simulink library "SimFly_Sensors"  (R2015b)
settings: Solver=VariableStepAuto  StartTime=0.0  StopTime=10.0  RelTol=1e-3
(part 1 of 2)
settings Model: Creator=mocherma  LastModifiedBy=mocherma

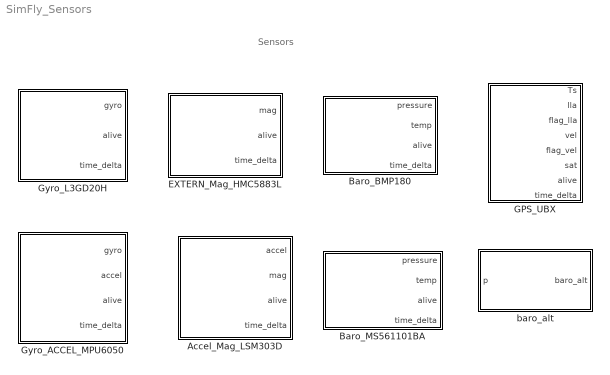
== system SimFly_Sensors ==
  note: Sensors
  Accel_Mag_LSM303D : MATLAB Function  TreatAsAtomicUnit=on  mask(SimFly Accel Magnetometer){sA0=HIGH, ascale=2G, lowPassFreq=773Hz, mscale=-/+ 2 gauss, rate=50Hz, lsm303d_sample_time=-1}
      mask prompts: ascale "Accel Scale"; lowPassFreq "Low Pass Cut-Off Frequency"; mscale "Mag Scale"; rate "Output Rate"; lsm303d_sample_time "SampleTime"
      mask help:
      | LSM303 MEMS motion sensor: 3-axis accelerometer and 3-axis magnetometer
      | Accelerometer full-scale range of ±2 g/±4 g/±8 g
      | Magnetometer ±1.3 to ±8,1 gauss magnetic field full-scale
      |
      | ...........Caution!................
      |
      | If External Magnetometer HMC5883L is in use SA0 must be
      |
      | HIGH due to the same I2C Address.
      |
      | ....................
      |
      | All quantities are in body axes. Signs are as follows:
      | +ax [rad/s]
      | +ay [rad/s]
      | +az [rad/s]
      | +mx [gauss]
      | +my [gauss]
      | +mz [gauss]
      |
      | Inputs are to pass through data when in simulation mode.
      | They are not used when model is deployed to hardware.
      |
      | Execution Time: 465 µS
      mask init:
      | sA0;
      | blk = gcb;
      | sA0String = get_param(blk,'sA0');
      | if strcmp(sA0String,'HIGH');
      |     sA0Pin = true;
      | else sA0Pin = false;
      | end
      | 
      | scaleaccString =get_param(blk,'ascale');
      | switch scaleaccString
      |     case '2G'
      |         scaleAc= uint8(0);
      |     case '4G'
      |         scaleAc= uint8(1);
      |     case '6G'
      |         scaleAc= uint8(2);
      |     case '8G'
      |         scaleAc= uint8(3);
      |     case '16G'
      |         scaleAc= uint8(4);
      |     otherwise
      |         scaleAc= uint8(0);
      | end
      | scalemagString =get_param(blk,'mscale');
      | switch scalemagString
      |     case '-/+ 2 gauss'
      |         scaleMag= uint8(0);
      |     case '-/+ 4 gauss'
      |         scaleMag= uint8(1);
      |     case '-/+ 8 gauss'
      |         scaleMag= uint8(2);
      |     case '-/+ 12 gauss'
      |         scaleMag= uint8(3);    
      |     otherwise
      |         scaleMag= uint8(1);
      | end        
      | lowPassString =get_param(blk,'lowPassFreq');
      | switch lowPassString
      |     case '773Hz'
      |         lowPassFreq= uint8(0);
      |     case '362Hz'
      |         lowPassFreq= uint8(1);
      |     case '194Hz'
      |         lowPassFreq= uint8(2);
      |     case '50Hz'
      |         lowPassFreq= uint8(3);    
      |     otherwise
      |         lowPassFreq= uint8(0);
      | end        
      | rateString =get_param(blk,'rate');
      | switch rateString
      |     case '50Hz'
      |         rateVal= uint8(0);
      |     case '100Hz'
      |         rateVal= uint8(1);
      |     case '200Hz'
      |         rateVal= uint8(2);
      |     case '400Hz'
      |         rateVal= uint8(3);
      |     otherwise
      |         rateVal= uint8(3);
      | end
  Baro_BMP180 : MATLAB Function  TreatAsAtomicUnit=on  mask(SimFly Barometer){osr=4.5ms, bmp180_sample_time=-1}
      mask prompts: osr "Oversampling Time"; bmp180_sample_time "Sample Time"
      mask help:
      | BMP180 DIGITAL PRESSURE SENSOR
      | Measures Pressure (mb)
      | Signs are as follows:
      | +p [mb]
      |
      | Oversampling Ratio: delay time for sampling measurements
      | 4.5ms / 7.5ms / 13.5ms / 25.5ms
      |
      | ........Caution......
      |
      | If used with Baro_MS5611 Baros's SD0 must be High
      |
      | .....................
      |
      |
      | Inputs are to pass through data when in simulation mode.
      | They are not used when model is deployed to hardware.
      |
      | Execution Time: 350µS
      mask init:
      | blk = gcb;
      | scaleString =get_param(blk,'osr');
      | switch scaleString
      |     case '4.5ms'
      |         osrValue= uint8(0);
      |     case '7.5ms'
      |         osrValue= uint8(1);
      |     case '13.5ms'
      |         osrValue= uint8(2);
      |     case '25.5ms'
      |         osrValue= uint8(3);        
      |     otherwise
      |         osrValue= uint8(0);
      | end
  Baro_MS561101BA : MATLAB Function  TreatAsAtomicUnit=on  mask(SimFly Barometer){sD0=LOW, osr=256, ms5611_sample_time=-1}
      mask prompts: osr "Oversampling Ratio"; ms5611_sample_time "Sample Time"
      mask help:
      | MS5611 DIGITAL PRESSURE SENSOR
      | Measures Pressure (mb)
      |
      | ...........Caution!................
      |
      | If  BMP180 is in use SD0 must be
      |
      | HIGH due to the same I2C Address.
      |
      | ...................................
      |
      |
      | Oversampling Ratio: delay time for sampling measurements
      | 256     =   1ms
      | 512     =   2ms
      | 1024    =   3ms
      | 2048    =   5ms
      | 4096    =   10ms
      |
      | Signs are as follows:
      | +p [mb]
      |
      | Inputs are to pass through data when in simulation mode.
      | They are not used when model is deployed to hardware.
      |
      | Execution Time: 600µS
      mask init:
      | sD0;
      | blk = gcb;
      | sD0String = get_param(blk,'sD0');
      | if strcmp(sD0String,'HIGH');
      |     sD0Pin = true;
      | else sD0Pin = false;
      | end
      | 
      | scaleString =get_param(blk,'osr');
      | switch scaleString
      |     case '256'
      |         osrValue= uint8(0);
      |     case '512'
      |         osrValue= uint8(1);
      |     case '1024'
      |         osrValue= uint8(2);
      |     case '2048'
      |         osrValue= uint8(3);
      |     case '4096'
      |         osrValue= uint8(4);          
      |     otherwise
      |         osrValue= uint8(1);
      | end
  EXTERN_Mag_HMC5883L : MATLAB Function  TreatAsAtomicUnit=on  mask(SimFly Magnetometer){range=+/- 0.88 Ga, rate=0.75Hz, samples=1, hmc_sample_time=-1}
      mask prompts: range "Sensor Field Range"; rate "Data Output Rate (Hz)"; samples "Number of samples averaged"; hmc_sample_time "Sample Time"
      mask help:
      | Honeywell HMC5883L MEMS 3-Axis Digital Compass
      | Magnetometer ±0.88 to ±8,1 gauss magnetic field full-scale
      | Output rate from 0.75Hz to 75Hz
      | Select number of samples averaged (1 to 8) per measurement output.
      |
      | ........Caution......
      |
      | If used with Accel LSM303 Accels's AD0 must be High
      |
      | .....................
      |
      | Inputs are to pass through data when in simulation mode.
      | They are not used when model is deployed to hardware.
      |
      | Execution Time: 555 µS
      mask init:
      | blk = gcb;
      | 
      | rangeString = get_param(blk,'range');
      | switch rangeString
      |     case '+/- 0.88 Ga'
      |         rangeString= uint8(1);
      |     case '+/-   1.3 Ga'
      |         rangeString= uint8(2);
      |     case '+/-   1.9 Ga'
      |         rangeString= uint8(3);
      |     case '+/-   2.5 Ga'
      |         rangeString= uint8(4);
      |     case '+/-   4.0 Ga'
      |         rangeString= uint8(5);
      |     case '+/-   4.7 Ga'
      |         rangeString= uint8(6);
      |     case '+/-   5.6 Ga'
      |         rangeString= uint8(7);
      |     case '+/-   8.1 Ga'
      |         rangeString= uint8(8);
      |     otherwise
      |         rangeString= uint8(1);
      | end
      | 
      | rateString =get_param(blk,'rate');
      | switch rateString
      |     case '0.75Hz'
      |         rateString= uint8(0);
      |     case '1.5Hz'
      |         rateString= uint8(1);
      |     case '3Hz'
      |         rateString= uint8(2);
      |     case '7.5Hz'
      |         rateString= uint8(3);
      |     case '15Hz'
      |         rateString= uint8(4);
      |     case '30Hz'
      |         rateString= uint8(5);
      |     case '75Hz'
      |         rateString= uint8(6);
      |     otherwise
      |         rateString= uint8(4);
      | end
      | 
      | 
      | samplesString =get_param(blk,'samples');
      | switch samplesString
      |     case '1'
      |         samplesString= uint8(0);
      |     case '2'
      |         samplesString= uint8(1);
      |     case '4'
      |         samplesString= uint8(2);
      |     case '8'
      |         samplesString= uint8(3);
      |     otherwise
      |         samplesString= uint8(0);
      | end
  GPS_UBX : MATLAB Function  TreatAsAtomicUnit=on  mask(SimFly GNSS){ubx_sample_time=-1}
      mask prompts: ubx_sample_time "Sample Time"
      mask help:
      | Block for parsing UMX data streams provided by GPS modules from Ublox.
      |
      | If using LEA-6H:
      | Max. Navigation update rate 5Hz
      |
      |
      | Ouput:
      | - Timestamp
      | - Latitude / Longitude [deg] / Altitude [m]
      | - LLA update flag
      | - ECEF velocity [m/s]
      | - vel update flag
      | - Number of visible satelites
      | - Alive flag
      | - Execution time
  Gyro_ACCEL_MPU6050 : MATLAB Function  TreatAsAtomicUnit=on  mask(SimFly IMU){AD0=HIGH, rate=50Hz, freqMp=5Hz, scaleAcc=2G, scaleGy=250DPS, mpuSampleTime=-1}
      mask prompts: rate "Output Rate"; freqMp "Lowpass Filter Cut Off Freq"; scaleAcc "Accel Scale"; scaleGy "Gyro Scale"; mpuSampleTime "Sample Time"
      mask help:
      | MPU-6050 device combines a 3-axis gyroscope and a 3-axis accelerometer
      | Gyro full-scale range of ±250, ±500, ±1000, and ±2000°/sec
      | Accelerometer full-scale range of ±2g, ±4g, ±8g, and ±16g.
      | All quantities are in body axes. Signs are as follows:
      | +p [rad/s]
      | +q [rad/s]
      | +r [rad/s]
      | +ax [m/s^2]
      | +ay [m/s^2]
      | +az [m/s^2]
      |
      | Inputs are to pass through data when in simulation mode.
      | They are not used when model is deployed to hardware.
      |
      | Execution Time: 464 µS
      mask init:
      | blk = gcb;
      | AD0;
      | AD0String = get_param(blk,'AD0');
      | if strcmp(AD0String,'HIGH');
      |     AD0Pin = true;
      | else AD0Pin = false;
      | end
      | scaleAccel =get_param(blk,'scaleAcc');
      | switch scaleAccel
      |     case '2G'
      |         scaleAccel= uint8(2);
      |     case '4G'
      |         scaleAccel= uint8(4);
      |     case '8G'
      |         scaleAccel= uint8(8);
      |     case '16G'
      |         scaleAccel= uint8(16);
      |     otherwise
      |         scaleAccel= uint8(2);
      | end
      | freqMpu =get_param(blk,'freqMp');
      | switch freqMpu
      |     case '5Hz'
      |         freqMpu= uint8(6);
      |     case '10Hz'
      |         freqMpu= uint8(5);
      |     case '21Hz'
      |         freqMpu= uint8(4);
      |     case '44Hz'
      |         freqMpu= uint8(3);
      |     case '94Hz'
      |         freqMpu= uint8(2);
      |     case '184Hz'
      |         freqMpu= uint8(1);
      |     otherwise
      |         freqMpu= uint8(1);
      | end    
      | 
      | scaleGyro =get_param(blk,'scaleGy');
      | switch scaleGyro
      |     case '250DPS'
      |         scaleGyro= int16(250);
      |     case '500DPS'
      |         scaleGyro= int16(500);
      |     case '1000DPS'
      |         scaleGyro= int16(1000);
      |     case '2000DPS'
      |         scaleGyro= int16(2000);
      |     otherwise
      |         scaleGyro= int16(250);
      | end  
      | 
      | rateString =get_param(blk,'rate');
      | switch rateString
      |     case '50Hz'
      |         rateVal= uint8(19);
      |     case '100Hz'
      |         rateVal= uint8(5);
      |     case '200Hz'
      |         rateVal= uint8(4);
      |     case '250Hz'
      |         rateVal= uint8(3);
      |     case '500Hz'
      |         rateVal= uint8(1);
      |     otherwise
      |         rateVal= uint8(3);
      | end
  Gyro_L3GD20H : MATLAB Function  TreatAsAtomicUnit=on  mask(SimFly Gyro){sD0=HIGH, scale=250DPS, freq=100Hz 12.5 Cut-Off[Hz], l3gd20_sampletime=-1}
      mask prompts: freq "Output Rate + Cutoff Freq"; l3gd20_sampletime "Sample Time"
      mask help:
      | L3GD20 MEMS motion sensor: 3-axis digital gyroscope
      | Gyro full-scale range of ±250, ±500 and ±2000°/sec
      | All quantities are in body axes. Signs are as follows:
      | +p [rad/s]
      | +q [rad/s]
      | +r [rad/s]
      |
      | Inputs are to pass through data when in simulation mode.
      | They are not used when model is deployed to hardware.
      |
      | Execution Time: 234 µS
      mask init:
      | sD0;
      | blk = gcb;
      | sD0String = get_param(blk,'sD0');
      | if strcmp(sD0String,'HIGH');
      |     sD0Pin = true;
      | else sD0Pin = false;
      | end
      | 
      | scaleString =get_param(blk,'scale');
      | switch scaleString
      |     case '250DPS'
      |         scaleValue= uint8(0);
      |     case '500DPS'
      |         scaleValue= uint8(1);
      |     case '2000DPS'
      |         scaleValue= uint8(2);
      |     otherwise
      |         scaleValue= uint8(1);
      | end
      | 
      | freqString =get_param(blk,'freq');
      | switch scaleString
      |     case '100Hz 12.5 Cut-Off[Hz]'
      |         freqValue= uint8(0);
      |     case '100Hz 25 Cut-Off[Hz]'
      |         freqValue= uint8(1);
      |     case '200Hz 0 Cut-Off[Hz]'
      |         freqValue= uint8(2);
      |     case '200Hz 12.5 Cut-Off[Hz]'
      |         freqValue= uint8(3);
      |     case '200Hz 70 Cut-Off[Hz]'
      |         freqValue= uint8(4);
      |     case '400Hz 20 Cut-Off[Hz]'
      |         freqValue= uint8(5);
      |     case '400Hz 50 Cut-Off[Hz]'
      |         freqValue= uint8(6);
      |     case '400Hz 110 Cut-Off[Hz]'
      |         freqValue= uint8(7);
      |     case '800Hz 30 Cut-Off[Hz]'
      |         freqValue= uint8(8);
      |     case '800Hz 100 Cut-Off[Hz]'
      |         freqValue= uint8(9);
      |     otherwise
      |         freqValue= uint8(2);    
      | end
  baro_alt : MATLAB Function  TreatAsAtomicUnit=on  mask(SimFly Barometer Altitude){p0=1013.25, alt_sample_time=-1}
      mask prompts: p0 "Pressure sea level"; alt_sample_time "Sample Time"
      mask help: Calculates the altitude above sea level with a given pressure at sea level in hPa

== matlab function SimFly_Sensors/Gyro_ACCEL_MPU6050 ==
  settings: updateMethod=DISCRETE  sampleTime=mpuSampleTime
  data: gyro output; accel output; alive output; time_delta output; AD0Pin parameter; freqMpu parameter; rateVal parameter; scaleGyro parameter; scaleAccel parameter
function [gyro,accel,alive,time_delta] = MPU6050(  AD0Pin, freqMpu, rateVal, scaleGyro, scaleAccel)
% Simulink Arduino Block Driver Library for Autocode Generation
 % 
 % This file is part of the Simulink Arduino Block Driver Library 
 % for Autocode Generation with Simulink
 %
 % This Library is free software: you can redistribute it and/or modify
 % it under the terms of the GNU General Public License as published by
 % the Free Software Foundation, either version 3 of the License, or
 % (at your option) any later version.
 %
 % This Library is distributed in the hope that it will be useful,
 % but WITHOUT ANY WARRANTY; without even the implied warranty of
 % MERCHANTABILITY or FITNESS FOR A PARTICULAR PURPOSE.  See the
 % GNU General Public License for more details.
 %
 % You should have received a copy of the GNU General Public License
 % along with this Library.  If not, see
 % <http://www.gnu.org/licenses/>.
 %
%
%PURMPOSE: Driver for MPU6050 with hardware abstraction layer
%AUTHOR: Marcell Mocher
%DATE: 10.6.2016
%VERSION: 0.1 V Fist build
%Input: -
%Output:    gyro[3*1](single) =  angular rates in X,Y,Z Axis [rad/s]
%           accel[3*1](single) = acceleration in X,Y,Z Axis [ms^-2]
%           alive(boolean) = boolean if sensor is alive
%           time_delta(single) = time needed to execute funtion [us]
%Info: This drive requires function call triggered simuluink functions in
% order to work
%Requires:  _get_time
%           _serial_init
%           _serial_print
%           _serial_write
%           _i2c_write_register
%           _i2c_read_register

persistent init_flag alive_flag MPU6050_ADDR gyroRes accelRes MPU6050_WHO_AM_I MPU6050_PWR_MGMT_1 MPU6050_CONFIG MPU6050_SMPLRT_DIV ...
    MPU6050_INT_ENABLE MPU6050_GYRO_CONFIG MPU6050_ACCEL_CONFIG MPU6050_GYRO_XOUT_H MPU6050_ACCEL_XOUT_H MPU6050_INT_PIN_CFG;


if strcmp(coder.target, 'rtw'),
    
    time_start = uint32(0);
    time_start = coder.ceval('_get_time');
    
    gyro = single(zeros(3,1));
    accel = single(zeros(3,1));
    
    %Parameter from Mask!
    debug = false;
    
    ad0 = AD0Pin;
    bandwidth = freqMpu;
    rate = rateVal;
    gyroScale = scaleGyro;
    acclScale = scaleAccel;
    
    if isempty(init_flag)
        
        init_flag = 1;
        
        %Init funtions
        coder.ceval('_delay_us',uint32(1000));
        coder.ceval('_i2c_init');
        coder.ceval('_delay_us',uint32(1000));
        
        if debug == true
            coder.ceval('_serial_init',uint32(250000));
        end
        
        % Calculate resolution
        gyroRes = (single(gyroScale)/32768.0)* pi/180;
        accelRes = (single(acclScale)/32768.0) * 9.80665;
        
        MPU6050_WHO_AM_I = uint8(hex2dec('75')); % Who AM I Register
        MPU6050_PWR_MGMT_1 = uint8(hex2dec('6B')); % Device defaults to the SLEEP mode
        MPU6050_CONFIG = uint8(hex2dec('1A'));
        MPU6050_SMPLRT_DIV = uint8(hex2dec('19'));
        MPU6050_INT_PIN_CFG = uint8(hex2dec('37'));
        MPU6050_INT_ENABLE = uint8(hex2dec('38'));
        MPU6050_GYRO_CONFIG = uint8(hex2dec('1B'));
        MPU6050_ACCEL_CONFIG = uint8(hex2dec('1C'));
        MPU6050_GYRO_XOUT_H = uint8(hex2dec('43'));
        MPU6050_ACCEL_XOUT_H = uint8(hex2dec('3B'));
        
        % Assign MPU AD0 status
        if ad0 == true
            MPU6050_ADDR = uint8(hex2dec('69')); % High Address
        else
            MPU6050_ADDR = uint8(hex2dec('68')); % Low Address
        end
        
        coder.ceval('_delay_us',uint32(1000));
        % Clear sleep mode bit (6), enable all sensors,  Set clock source to be PLL with x-axis gyroscope reference, bits 2:0 = 001
        coder.ceval('_i2c_write_register',MPU6050_ADDR,MPU6050_PWR_MGMT_1,uint8(1));
        
        %Check if sensor is connected
        val = uint8(zeros(6,1));
        coder.ceval('_i2c_read_register',MPU6050_ADDR,MPU6050_WHO_AM_I,uint8(1),coder.ref(val));
        
        if uint8(hex2dec('68')) == val(1)
            alive_flag = true;
        else
            alive_flag = false;
        end
        
        % Configure Gyro and Accelerometer
        % Disable FSYNC and set accelerometer and gyro bandwidth to 44 and 42 Hz, respectively;
        % DLPF_CFG = bits 2:0 = 010; this sets the sample rate at 1 kHz for both
        % Maximum delay time is 4.9 ms corresponding to just over 200 Hz sample rate
        % bandwith 1 = 184Hz
        % bandwith 2 = 94Hz
        % bandwith 3 = 44Hz
        % bandwith 4 = 21Hz
        % bandwith 5 = 10Hz
        % bandwith 6 = 5Hz
        coder.ceval('_i2c_write_register',MPU6050_ADDR,MPU6050_CONFIG,uint8(bandwidth));
        
        % Set sample rate = gyroscope output rate/(1 + SMPLRT_DIV), Use a 500 Hz rate;
        % rate 1 = 500Hz
        % rate 3 = 250Hz
        % rate 4 = 200Hz
        % rate 5 = 100Hz
        % rate 19 = 50Hz
        coder.ceval('_i2c_write_register',MPU6050_ADDR, MPU6050_SMPLRT_DIV,uint8(rate));
        
        % enable I2C_BYPASS_EN so additional chips can join the I2C bus and all can be controlled by the Arduino as master
        coder.ceval('_i2c_write_register',MPU6050_ADDR, MPU6050_INT_PIN_CFG, uint8(34));
        
        % Enable data ready (bit 0) interrupt
        
        coder.ceval('_i2c_write_register',MPU6050_ADDR, MPU6050_INT_ENABLE, uint8(1));
        
        % Set gyroscope scale
        % 0 = 250 DPS
        % 8 = 500 DPS
        % 16 = 1000 DPS
        % 24 = 2000 DPS
        switch gyroScale
            case 250
                res_val = uint8(0);
            case 500
                res_val = uint8(8);
            case 1000
                res_val = uint8(16);
            case 2000
                res_val = uint8(24);
        end
        coder.ceval('_i2c_write_register',MPU6050_ADDR, MPU6050_GYRO_CONFIG, res_val);
        
        % Set gyroscope scale
        % 0 = 2 G
        % 8 = 4 g
        % 16 = 8G
        % 24 = 16G
        switch acclScale
            case 2
                res_val = uint8(0);
            case 4
                res_val = uint8(8);
            case 8
                res_val = uint8(16);
            case 16
                res_val = uint8(24);
        end
        coder.ceval('_i2c_write_register',MPU6050_ADDR, MPU6050_ACCEL_CONFIG, res_val);
    end
    
    % Read Gyro Register
    if alive_flag == true
        
    val = uint8(zeros(6,1));
    coder.ceval('_i2c_read_register',MPU6050_ADDR,MPU6050_GYRO_XOUT_H,uint8(6),coder.ref(val));
    gyro(1) = single(typecast([val(2) val(1)],'int16')) * gyroRes;
    gyro(2) = -single(typecast([val(4) val(3)],'int16')) * gyroRes;
    gyro(3) = -single(typecast([val(6) val(5)],'int16')) * gyroRes;
    
    
    % Read Accel Register
    val = uint8(zeros(6,1));
    coder.ceval('_i2c_read_register',MPU6050_ADDR,MPU6050_ACCEL_XOUT_H,uint8(6),coder.ref(val));
    accel(1) = -single(typecast([val(2) val(1)],'int16')) * accelRes;
    accel(2) = single(typecast([val(4) val(3)],'int16')) * accelRes;
    accel(3) = single(typecast([val(6) val(5)],'int16')) * accelRes;
    
    else
        
    gyro = single(zeros(3,1));
    accel = single(zeros(3,1));    
        
    end
    

    time_end = uint32(0);
    time_end = coder.ceval('_get_time');
    time_delta = time_end - time_start;
    alive = alive_flag;
    
else
    gyro = single(zeros(3,1));
    accel = single(zeros(3,1));
    alive = true;
    time_delta = uint32(1);
end



end

== matlab function SimFly_Sensors/Accel_Mag_LSM303D ==
  settings: updateMethod=DISCRETE  sampleTime=lsm303d_sample_time
  data: accel output; mag output; alive output; time_delta output; sA0Pin parameter; scaleAc parameter; scaleMag parameter; lowPassFreq parameter; rateVal parameter
function [accel,mag,alive,time_delta] = LSM303D(sA0Pin, scaleAc, scaleMag, lowPassFreq, rateVal)
% Simulink Arduino Block Driver Library for Autocode Generation
 % 
 % This file is part of the Simulink Arduino Block Driver Library 
 % for Autocode Generation with Simulink
 %
 % This Library is free software: you can redistribute it and/or modify
 % it under the terms of the GNU General Public License as published by
 % the Free Software Foundation, either version 3 of the License, or
 % (at your option) any later version.
 %
 % This Library is distributed in the hope that it will be useful,
 % but WITHOUT ANY WARRANTY; without even the implied warranty of
 % MERCHANTABILITY or FITNESS FOR A PARTICULAR PURPOSE.  See the
 % GNU General Public License for more details.
 %
 % You should have received a copy of the GNU General Public License
 % along with this Library.  If not, see
 % <http://www.gnu.org/licenses/>.
 %
%
%PURMPOSE: Driver for LSM303D with hardware abstraction layer
%AUTHOR: Marcell Mocher
%DATE: 11.6.2016
%VERSION: 0.1V Fist build
%Input: -
%Output:    accel[3*1](single) = acceleration in X,Y,Z Axis [ms^-2]
%           mag[3*1](single) = magnetic field in X,Y,Z Axis [gauss]
%           alive(boolean) = boolean if sensor is alive
%           time_delta(single) = time needed to execute funtion [us]
%Info: This drive requires function call triggered simuluink functions in
% order to work
%Requires:  _get_time
%           _serial_init
%           _serial_print
%           _serial_write
%           _i2c_write_register
%           _i2c_read_register

persistent init_flag alive_flag LSM303D_ADDR LSM303_CTRL1 LSM303_CTRL2 LSM303_CTRL5 LSM303_CTRL6 LSM303_CTRL7...
    accel_MG_LSB magGauss_LSB

if strcmp(coder.target, 'rtw'),
    
    time_start = uint32(0);
    time_start = coder.ceval('_get_time');
    
    %Parameter from Mask!
    sa0 = sA0Pin;
    rate = rateVal;
    scale_accel = scaleAc;
    low_pass_freq = lowPassFreq;
    scale_mag = scaleMag;
    
    if isempty(init_flag)
        init_flag = 0;
        alive_flag = false;
        accel = single(zeros(3,1));
        mag = single(zeros(3,1));
        LSM303_CTRL1 = uint8(hex2dec('20'));
        LSM303_CTRL2 = uint8(hex2dec('21'));
        LSM303_CTRL5 = uint8(hex2dec('24'));
        LSM303_CTRL6 = uint8(hex2dec('25'));
        LSM303_CTRL7 = uint8(hex2dec('26'));
        
        % Init functions
        coder.ceval('_i2c_init');
        
        % Assign MPU SA0 status
        if sa0 == true
            LSM303D_ADDR = uint8(29); % High Address
        else
            LSM303D_ADDR = uint8(30); % Low Address
        end
        
        
        
        switch rate
            case 0 % 50 Hz
                ctrl1_odr = uint8(hex2dec('57'));
                
            case 1 % 100 Hz
                ctrl1_odr = uint8(hex2dec('67'));
                
            case 2 % 200 Hz
                ctrl1_odr = uint8(hex2dec('77'));
                
            case 3 % 400 Hz
                ctrl1_odr = uint8(hex2dec('87'));
            otherwise
                ctrl1_odr = uint8(hex2dec('87'));
        end
        
        %Set sampling rate
        coder.ceval('_i2c_write_register',LSM303D_ADDR,LSM303_CTRL1,uint8(ctrl1_odr));
        
        
        %Check if enabling has worked for accel
        val = uint8(zeros(6,1));
        coder.ceval('_i2c_read_register',LSM303D_ADDR,LSM303_CTRL1,uint8(1),coder.ref(val));
        if  val(1) == ctrl1_odr
            alive_flag = true;
        end
        
        
        % Register 2 % Set scale for Accel and Filter Mode
        %
        %Filter low pass
        % 00 773 Hz = 0x00 % Default
        % 01 194 Hz = 0x40
        % 10 362 Hz = 0x80
        % 11  50 Hz = 0xC0
        %Accel Scale
        % 000  2g    % Default
        % 001  4g
        % 010  6g
        % 011  8g
        % 100 16g
        %
        %Register Value: Filter + Accel
        %
        switch scale_accel
            case 0 % +/- 2g
                ctrl2_scale_acc = uint8(hex2dec('00'));
                accel_MG_LSB = single(0.000061 * 9.80665); % mg per lsb
                
            case 1 % +/- 4g
                ctrl2_scale_acc = uint8(hex2dec('08'));
                accel_MG_LSB = single(0.000122 * 9.80665); % mg per lsb
                
            case 2 % +/- 6g
                ctrl2_scale_acc = uint8(hex2dec('10'));
                accel_MG_LSB = single(0.000183 * 9.80665); % mg per lsb
                
            case 3 % +/- 8g
                ctrl2_scale_acc = uint8(hex2dec('18'));
                accel_MG_LSB = single(0.000244 * 9.80665); % mg per lsb
                
            case 4 % +/- 16g
                ctrl2_scale_acc = uint8(hex2dec('20'));
                accel_MG_LSB = single(0.000732 * 9.80665); % mg per lsb
                
            otherwise
                ctrl2_scale_acc = uint8(hex2dec('00'));
                accel_MG_LSB = single(0.000061 * 9.80665); % mg per lsb
        end
        
        switch low_pass_freq
            case 0 % 773 Hz
                ctrl2_lowpass_acc = uint8(hex2dec('00'));
                
            case 1 % 362 Hz
                ctrl2_lowpass_acc = uint8(hex2dec('80'));
                
            case 2 % 194 Hz
                ctrl2_lowpass_acc = uint8(hex2dec('40'));
                
            case 3 % 50 Hz
                ctrl2_lowpass_acc = uint8(hex2dec('C0'));
                
            otherwise% 773 Hz
                ctrl2_lowpass_acc = uint8(hex2dec('00'));
        end
        
        ctrl2_reg = ctrl2_scale_acc + ctrl2_lowpass_acc;
        coder.ceval('_i2c_write_register',LSM303D_ADDR,LSM303_CTRL2,uint8(ctrl2_reg));
        % Enable the magnetometer :
        % 0x74 = 0b01110100
        % M_RES = 11 (high resolution mode); M_ODR = 101 (100 Hz ODR)
        coder.ceval('_i2c_write_register',LSM303D_ADDR,LSM303_CTRL5,uint8(hex2dec('74')));
        
        %Check if mag is responding
        % Register 6 % Set scale for Mag
        %Register Value: 0 + Mag + 00000
        %2G  = 0x00;
        %4G  = 0x20;
        %8G  = 0x40;
        %12G = 0x60;
        
        switch scale_mag
            
            case 0 % 2 gauss
                magGauss_LSB = single(0.000080); % gauss/LSB
                coder.ceval('_i2c_write_register',LSM303D_ADDR,LSM303_CTRL6,uint8(hex2dec('00')));
            case 1 % 4 gauss
                magGauss_LSB = single(0.000160);
                coder.ceval('_i2c_write_register',LSM303D_ADDR,LSM303_CTRL6,uint8(hex2dec('20')));
            case 2 % 8 gauss
                magGauss_LSB = single(0.000320);
                coder.ceval('_i2c_write_register',MPU6050_ADDR,LSM303D_ADDR,LSM303_CTRL6,uint8(hex2dec('40')));
            case 3 % 12 gauss
                magGauss_LSB = single(0.000479);
                coder.ceval('_i2c_write_register',LSM303D_ADDR,LSM303_CTRL6,uint8(hex2dec('60')));
            otherwise
                magGauss_LSB = single(0.000080);
                coder.ceval('_i2c_write_register',LSM303D_ADDR,LSM303_CTRL6,uint8(hex2dec('00')));
        end
        
        % 0x00 = 0b00000000
        % MLP = 0 (low power mode off); MD = 00 (continuous-conversion mode)
        coder.ceval('_i2c_write_register',LSM303D_ADDR,LSM303_CTRL7,uint8(hex2dec('00')));
    end
    
    if alive_flag == true
        
        val = uint8(zeros(6,1));
        coder.ceval('_i2c_read_register',LSM303D_ADDR,uint8(168),uint8(6),coder.ref(val));
        accel(1) = single(typecast([val(1) val(2)],'int16'))* accel_MG_LSB;
        accel(2) = -single(typecast([val(3) val(4)],'int16'))* accel_MG_LSB;
        accel(3) = single(typecast([val(5) val(6)],'int16'))* accel_MG_LSB;
        
        val = uint8(zeros(6,1));
        coder.ceval('_i2c_read_register',LSM303D_ADDR,uint8(136),uint8(6),coder.ref(val));
        mag(1) = -single(typecast([val(1) val(2)],'int16'))* magGauss_LSB; %-
        mag(2) = single(typecast([val(3) val(4)],'int16'))* magGauss_LSB;
        mag(3) = -single(typecast([val(5) val(6)],'int16'))* magGauss_LSB; %-
        
    else
        
        accel = single(zeros(3,1));
        mag = single(zeros(3,1));
        
    end
    
    alive = alive_flag;
    time_end = uint32(0);
    time_end = coder.ceval('_get_time');
    time_delta = time_end - time_start;
    
    %Simulation mode only
else
    
    accel = single(zeros(3,1));
    mag = single(zeros(3,1));
    alive = true;
    time_delta = uint32(1);
end

== matlab function SimFly_Sensors/Baro_BMP180 ==
  settings: updateMethod=DISCRETE  sampleTime=bmp180_sample_time
  data: pressure output; temp output; alive output; time_delta output; osrValue parameter
function [ pressure,temp,alive,time_delta] = BMP180(osrValue)
% Simulink Arduino Block Driver Library for Autocode Generation
 % 
 % This file is part of the Simulink Arduino Block Driver Library 
 % for Autocode Generation with Simulink
 %
 % This Library is free software: you can redistribute it and/or modify
 % it under the terms of the GNU General Public License as published by
 % the Free Software Foundation, either version 3 of the License, or
 % (at your option) any later version.
 %
 % This Library is distributed in the hope that it will be useful,
 % but WITHOUT ANY WARRANTY; without even the implied warranty of
 % MERCHANTABILITY or FITNESS FOR A PARTICULAR PURPOSE.  See the
 % GNU General Public License for more details.
 %
 % You should have received a copy of the GNU General Public License
 % along with this Library.  If not, see
 % <http://www.gnu.org/licenses/>.
 %
%
%PURMPOSE: Driver for BMP180 with hardware abstraction layer
%AUTHOR: Marcell Mocher
%DATE: 11.6.2016
%VERSION: 0.1V Fist build
%Input: -
%Output:    pressure[1](single) = pressure [millibar]
%           temp[1](single) = temperature [°C]
%           alive(boolean) = boolean if sensor is alive
%           time_delta(single) = time needed to execute funtion [us]
%Info: This driver requires function call triggered simulink functions in
% order to work see requires
%Requires:  _get_time
%           _serial_init
%           _serial_print
%           _serial_write
%           _i2c_write_register
%           _i2c_read_register

persistent init_flag alive_flag delayOversampling startTimeTemp...
    startTimePress state BMP180_I2CADDR ac b m rawTemperature...
    bmpTemperature BMP180_CONTROL BMP180_TEMPDATA BMP180_PRESSUREDATA...
    BMP180_READTEMPCMD BMP180_READPRESSURECMD bmpPressure raw_press

if strcmp(coder.target, 'rtw'),
    
    time_start = uint32(0);
    time_start = coder.ceval('_get_time');
    
    %Parameter from Mask!
    oversampling = osrValue;
    
    if isempty(init_flag)
        init_flag = 0;
        alive_flag = false;
        startTimeTemp = uint32(0);
        startTimePress = uint32(0);
        state = uint8(0);
        rawTemperature = uint16(0);
        bmpTemperature = single(0);
        bmpPressure = int32(0);
        raw_press = uint32(0);
        BMP180_I2CADDR = uint8(hex2dec('77'));
        BMP180_CONTROL = uint8(hex2dec('F4'));
        BMP180_TEMPDATA = uint8(hex2dec('F6'));
        BMP180_PRESSUREDATA = uint8(hex2dec('F6'));
        BMP180_READTEMPCMD = uint8(hex2dec('2E'));
        BMP180_READPRESSURECMD = uint8(hex2dec('34'));
        
        % Init functions
        coder.ceval('_i2c_init');
        
        
        % Get oversampling delay
        switch oversampling
            case 0
                delayOversampling = uint32(4500);
            case 1
                delayOversampling = uint32(7500);
            case 2
                delayOversampling = uint32(13500);
            case 3
                delayOversampling = uint32(25500);
            otherwise
                delayOversampling = uint32(25500);
        end
        
        % Check if sensor is connected
        val = uint8(zeros(6,1));
        coder.ceval('_i2c_read_register',BMP180_I2CADDR,uint8(208),uint8(1),coder.ref(val));
        if val(1) == uint8(85)
            alive_flag = true;
        end
        
        % Read calibration data from registers
        BMP180_CAL_A = uint8([uint8(hex2dec('AA'));
            uint8(hex2dec('AC'));
            uint8(hex2dec('AE'));
            uint8(hex2dec('B0'));
            uint8(hex2dec('B2'));
            uint8(hex2dec('B4'))]);
        
        BMP180_CAL_B = uint8([uint8(hex2dec('B6'));
            uint8(hex2dec('B8'))]);
        
        BMP180_CAL_M = uint8([uint8(hex2dec('BA'));
            uint8(hex2dec('BC'));
            uint8(hex2dec('BE'))]);
        
        % Note: AC1 AC2 AC3 int16
        %       AC4 AC5 AC6 uint16
        ac = uint16(zeros(6,1));
        for i = 1:6
            val = uint8(zeros(6,1));
            coder.ceval('_i2c_read_register',BMP180_I2CADDR,BMP180_CAL_A(i),uint8(2),coder.ref(val));
            ac(i) = typecast([val(2) val(1)],'uint16');
        end
        
        b = int16(zeros(2,1));
        for i = 1:2
            val = uint8(zeros(6,1));
            coder.ceval('_i2c_read_register',BMP180_I2CADDR,BMP180_CAL_B(i),uint8(2),coder.ref(val));
            b(i) = typecast([val(2) val(1)],'int16');
        end
        
        m = int16(zeros(3,1));
        for i = 1:3
            val = uint8(zeros(6,1));
            coder.ceval('_i2c_read_register',BMP180_I2CADDR,BMP180_CAL_M(i),uint8(2),coder.ref(val));
            m(i) = typecast([val(2) val(1)],'int16');
            
        end
    end
    
    if alive_flag == true
        
    switch state
        case 0 % start temp reading
            coder.ceval('_i2c_write_register',BMP180_I2CADDR,BMP180_CONTROL,BMP180_READTEMPCMD);
            startTimeTemp = coder.ceval('_get_time');
            state = state + 1;
        case 1 % wait for 4.5ms and then read Raw Temperature
            time = uint32(0);
            time = coder.ceval('_get_time');
            if (time - startTimeTemp) > 4500
                val = uint8(zeros(6,1));
                coder.ceval('_i2c_read_register',BMP180_I2CADDR,BMP180_TEMPDATA,uint8(2),coder.ref(val));
                rawTemperature = typecast([val(2),val(1)],'uint16');
                bmpTemperature = calcTemperature(rawTemperature,ac,m);
                coder.ceval('_i2c_write_register',BMP180_I2CADDR,BMP180_CONTROL,BMP180_READPRESSURECMD+bitshift(oversampling,6)); % start press reading
                startTimePress = coder.ceval('_get_time');
                state = state + 1;
            end
        case 2 % wait for Oversampling time and then read Raw Temperature
            time = uint32(0);
            time = coder.ceval('_get_time');
            if (time - startTimePress) > delayOversampling
                val = uint8(zeros(6,1));
                val2 = uint8(zeros(6,1));
                coder.ceval('_i2c_read_register',BMP180_I2CADDR,BMP180_PRESSUREDATA,uint8(2),coder.ref(val));
                coder.ceval('_i2c_read_register',BMP180_I2CADDR,BMP180_PRESSUREDATA+2,uint8(1),coder.ref(val2));
                raw_press= typecast([val2(1),val(2),val(1),0],'uint32');
                raw_press = bitshift(raw_press,-(8-int8(oversampling)));
                bmpPressure = computePressure(raw_press,computeB5(rawTemperature,ac,m),ac,b,oversampling);
                state = uint8(0);
            end
        otherwise
            state = uint8(0);
    end
    end
    pressure = single(bmpPressure) * 0.01;   %PA to millibar
    temp = bmpTemperature;
    alive = alive_flag;
    
    time_end = uint32(0);
    time_end = coder.ceval('_get_time');
    time_delta = time_end - time_start;
    %for simulation only
else
    pressure = single(1);
    temp = single(1);
    alive = true;
    time_delta = uint32(1);
    
end

end

%Calculates the termperature according to Datasheet Page 15
function bmp_temp = calcTemperature(raw_temp,ac,m)
b5 = computeB5(raw_temp,ac,m);
bmp_temp = single(bitshift((b5 + 8),-4)) * 0.1;
end


% Calculates the value B5 according to Datasheet Page 15
function b5 = computeB5(raw_temp,ac,m)
X1 = int32(bitshift((int32(raw_temp) - int32(ac(6))) * int32(ac(5)),-15));
X2 = int32(bitshift(int32(m(2)),11) / (X1 + int32(m(3))));
b5 = int32(X1 + X2);
end

% Calculates the pressure according to Datasheet Page 15
function bmp_press = computePressure(raw_press,b5,ac,b,oversampling)

ac1 = typecast(ac(1),'int16');
ac2 = typecast(ac(2),'int16');
ac3 = typecast(ac(3),'int16');

B6 = int32(b5 - 4000);
X1 = int32(bitshift(int32(b(2)) * bitshift((B6 * B6),-12),-11));
X2 = int32(bitshift((int32(ac2) * B6),-11));
X3 = int32(X1 + X2);
B3 = int32(bitshift((bitshift((int32(ac1) * 4 + X3),oversampling) + 2),-2));
X1 = bitshift((int32(ac3) * B6),-13);
X2 = bitshift((int32(b(1)) * bitshift((B6 * B6),-12)),-16);
X3 = bitshift(((X1 + X2) + 2),-2);
B4 = uint32(bitshift((uint32(ac(4)) * uint32((X3 + 32768))),-15));
B7 = uint32((int32(raw_press) - B3) * bitshift(int32(50000), -oversampling));

if B7 < 2.1475e+09
    p = int32((bitshift(B7,1)) / B4);
else
    p = int32(bitshift((B7 / B4),1));
end

X1 = bitshift(p,-8) * bitshift(p,-8);
X1 = bitshift((X1 * 3038),-16);
X2 = bitshift((-7357 * p),-16);
bmp_press =  p + bitshift((X1 + X2 + int32(3791)),-4);

end

== matlab function SimFly_Sensors/EXTERN_Mag_HMC5883L ==
  settings: updateMethod=DISCRETE  sampleTime=hmc_sample_time
  data: mag output; alive output; time_delta output; rangeString parameter; rateString parameter; samplesString parameter
function [mag,alive,time_delta] = fcn(  rangeString, rateString, samplesString)
% Simulink Arduino Block Driver Library for Autocode Generation
 % 
 % This file is part of the Simulink Arduino Block Driver Library 
 % for Autocode Generation with Simulink
 %
 % This Library is free software: you can redistribute it and/or modify
 % it under the terms of the GNU General Public License as published by
 % the Free Software Foundation, either version 3 of the License, or
 % (at your option) any later version.
 %
 % This Library is distributed in the hope that it will be useful,
 % but WITHOUT ANY WARRANTY; without even the implied warranty of
 % MERCHANTABILITY or FITNESS FOR A PARTICULAR PURPOSE.  See the
 % GNU General Public License for more details.
 %
 % You should have received a copy of the GNU General Public License
 % along with this Library.  If not, see
 % <http://www.gnu.org/licenses/>.
 %
%
%PURPOSE: Driver for HMC5883L with hardware abstraction layer
%AUTHOR: Marcell Mocher
%DATE: 10.6.2016
%VERSION: 0.1 V Fist build
%Input: -
%Output:    gyro[3*1](single) =  angular rates in X,Y,Z Axis [rad/s]
%           accel[3*1](single) = acceleration in X,Y,Z Axis [ms^-2]
%           alive(boolean) = boolean if sensor is alive
%           time_delta(single) = time needed to execute funtion [us]
%Info: This drive requires function call triggered simuluink functions in
% order to work
%Requires:  _get_time
%           _serial_init
%           _serial_print
%           _serial_write
%           _i2c_write_register
%           _i2c_read_register
%           _delay_us



persistent init_flag alive_flag HMC5883L_ADDR gaussPerDigit...
    HMC5883L_REG_OUT_X_M HMC5883L_REG_OUT_Y_M HMC5883L_REG_OUT_Z_M

if strcmp(coder.target, 'rtw'),
    
    time_start = uint32(0);
    time_start = coder.ceval('_get_time');
    
    % Parameter from Mask!
    range = rangeString; % Define Range setting from 1 to 8
    rate = rateString; % Define outdate rate from 0 to 6
    samples = samplesString; % Define oversampling rate 0 to 3 [1 2 4 8 samples]

    % Init parameters
    mag = single((zeros(3,1)));
    
    if isempty(init_flag)
        init_flag = 0;
        alive_flag = false;
        gaussPerDigit = single(0);
        time_delta = uint32(1);
        alive =  false;
        HMC5883L_ADDR           = uint8(hex2dec('1E'));
        HMC5883L_REG_CONFIG_A	= uint8(hex2dec('00'));
        HMC5883L_REG_CONFIG_B	= uint8(hex2dec('01'));
        HMC5883L_REG_MODE       = uint8(hex2dec('02'));
        HMC5883L_REG_OUT_X_M	= uint8(hex2dec('03'));
        %HMC5883L_REG_OUT_X_L	= uint8(hex2dec('04'));
        HMC5883L_REG_OUT_Z_M	= uint8(hex2dec('05'));
        %HMC5883L_REG_OUT_Z_L	= uint8(hex2dec('06'));
        HMC5883L_REG_OUT_Y_M	= uint8(hex2dec('07'));
        %HMC5883L_REG_OUT_Y_L	= uint8(hex2dec('08'));
        %HMC5883L_REG_STATUS     = uint8(hex2dec('09'));
        HMC5883L_REG_IDENT_A	= uint8(hex2dec('0A'));
        HMC5883L_REG_IDENT_B	= uint8(hex2dec('0B'));
        HMC5883L_REG_IDENT_C	= uint8(hex2dec('0C'));
        HMC5883L_CONTINOUS     = uint8(0);
        
        % Init funtions
        coder.ceval('_i2c_init');
        
        % See if HMC5883L is responding
        id_a = uint8(0);
        coder.ceval('_i2c_read_register',HMC5883L_ADDR,HMC5883L_REG_IDENT_A,uint8(1),coder.ref(id_a));
        
        id_b = uint8(0);
        coder.ceval('_i2c_read_register',HMC5883L_ADDR,HMC5883L_REG_IDENT_B,uint8(1),coder.ref(id_b));
        
        id_c = uint8(0);
        coder.ceval('_i2c_read_register',HMC5883L_ADDR,HMC5883L_REG_IDENT_C,uint8(1),coder.ref(id_c));
        
        if (id_a(1) == uint8(72)) && (id_b(1) == uint8(52)) && (id_c(1) == uint8(51))
            alive_flag = true;
        else
            return;
        end
        
        % Set resolution  0.88Ga 1.3Ga 1.9Ga 2.5Ga 4.0Ga 4.7Ga 5.6Ga 8.1Ga
        resolution = single([0.73 0.92 1.22 1.52 2.27 2.56 3.03 4.35] * 1e-3) ;
        gaussPerDigit = resolution(range);
        coder.ceval('_i2c_write_register',HMC5883L_ADDR,HMC5883L_REG_CONFIG_B,bitshift((range-uint8(1)),5));
        % Set continous measurement mode
        %val = I2C_readRegister(HMC5883L_ADDR,HMC5883L_REG_MODE,uint8(1));
        %val(1) = bitand(val(1),uint8(bin2dec('11111100')));
        %val(1) = bitor(val(1),HMC5883L_CONTINOUS);
        coder.ceval('_i2c_write_register',HMC5883L_ADDR,HMC5883L_REG_MODE,HMC5883L_CONTINOUS);
        
        % Set data rate
        val = uint8(0);
        coder.ceval('_i2c_read_register',HMC5883L_ADDR,HMC5883L_REG_CONFIG_A,uint8(1),coder.ref(val));
        val(1) = bitand(val(1),uint8(bin2dec('11100011')));
        val(1) = bitor(val(1),bitshift(rate,2));
        coder.ceval('_i2c_write_register',HMC5883L_ADDR,HMC5883L_REG_CONFIG_A,val(1));
        % Set oversampling rate
        coder.ceval('_i2c_read_register',HMC5883L_ADDR,HMC5883L_REG_CONFIG_A,uint8(1),coder.ref(val));
        val(1) = bitand(val(1),uint8(bin2dec('10011111')));
        val(1) = bitor(val(1),bitshift(samples,5));
        coder.ceval('_i2c_write_register',HMC5883L_ADDR,HMC5883L_REG_CONFIG_A,val(1));

        % Test = get Samples
        %     val = I2C_readRegister(HMC5883L_ADDR,HMC5883L_REG_CONFIG_A,uint8(1));
        %     val(1) = bitand(val(1),uint8(bin2dec('01100000')));
        %     val(1) =bitshift(val(1),-5);
        %     stest = val(1);
        
    end
    
    % Only do readings if sensor is healthy
    if alive_flag == true
        val6 = uint8(zeros(6,1));
        coder.ceval('_i2c_read_register',HMC5883L_ADDR,HMC5883L_REG_OUT_X_M,uint8(6),coder.ref(val6));
        mag(2) = single(typecast([val6(2),val6(1)],'int16')) * gaussPerDigit;
        mag(3) = single(typecast([val6(4),val6(3)],'int16')) * gaussPerDigit;
        mag(1) = -single(typecast([val6(6),val6(5)],'int16')) * gaussPerDigit;
    end
    alive = alive_flag;
    time_end = uint32(0);
    time_end = coder.ceval('_get_time');
    time_delta = time_end - time_start;
    %for simulation only
else
    mag = single(zeros(3,1));
    alive = true;
    time_delta = uint32(1);
    
end

end
